simulink model "acc_vm"  (R2025b)
settings: Solver=FixedStepDiscrete  StartTime=0.0  StopTime=10.0  RelTol=1e-3
settings Model: Creator=matthewkeller  LastModifiedBy=ryanj
settings OptimizationCC: DefaultParameterBehavior=Inlined  EnhancedBackFolding=on  PassReuseOutputArgsThreshold=0.0  ZeroExternalMemoryAtStartup=off  ZeroInternalMemoryAtStartup=off  OptimizeBlockOrder=speed  DifferentSizesBufferReuse=on  OptimizationCustomize=off
settings DebuggingCC: ParameterTunabilityLossMsg=error
settings SFSimCC: MATLABDynamicMemAlloc=off
settings RTWCC: SystemTargetFile=rtmaps.tlc  TemplateMakefile=rtmaps_default_tmf  PostCodeGenCommand=rtmaps_post_code_generation(buildInfo)  RetainRTWFile=on  TargetLang=C++  Description=Generate an RTMaps component embedding the model
settings CodeAppCC: ForceParamTrailComments=on  OperatorAnnotations=on
settings STFCustomTargetCC: SystemTargetFile=rtmaps.tlc  TargetLangStandard=C++11 (ISO)  ModelReferenceCompliant=off  CombineOutputUpdateFcns=on  CodeInterfacePackaging=C++ class  SubcomponentCodeInterfacePackaging=C++ class  CPPClassGenCompliant=on  GRTInterface=off  CustomFileTemplate=rtmaps_file_process.tlc  RTMaps_CombineOutputUpdateFcns=1  RTMaps_MatFileLogging=0  DisplayOptimOptions=off  RTMAPS_SDKDIR=C:\Program Files\Intempora\RTMaps 4  RTMAPS_OS=vc.net2022  RTMaps_IntegerCode=0  RTMAPS_BOARD=vc.net2022_x64  RTMaps_GenerateAllocFcn=0  RTMaps_GenerateERTSFunction=0  RTMaps_GRTInterface=0  RTMaps_MultiInstanceCode=1  RTMAPS_ARCH=x86_64
settings GRTTargetCC: TargetLangStandard=C++11 (ISO)  ModelReferenceCompliant=off  ParMdlRefBuildCompliant=off  CompOptLevelCompliant=off  MatFileLogging=off  CodeInterfacePackaging=C++ class  SubcomponentCodeInterfacePackaging=C++ class  UseToolchainInfoCompliant=off

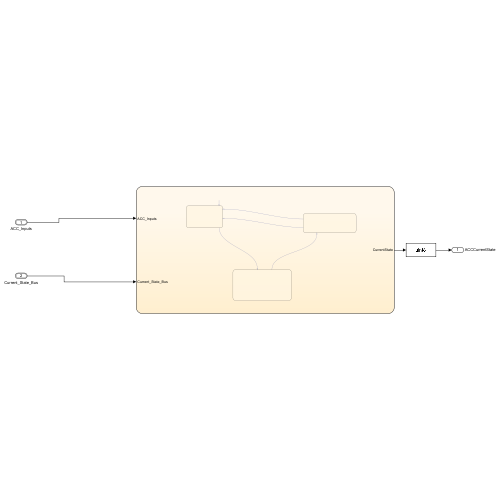
[thumbnail: Simulink's stored preview of the top-level diagram]
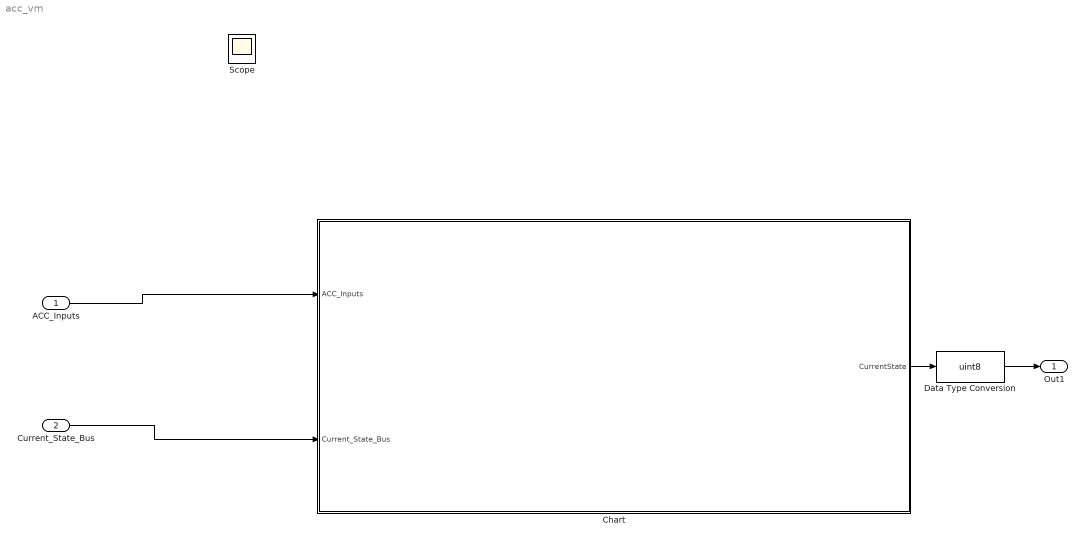
== system acc_vm ==
  ACC_Inputs : Inport  OutDataTypeStr=Bus: ACCStatusBus
  Current_State_Bus : Inport  Port=2  OutDataTypeStr=Bus: CurrentStateBus
  Chart : Stateflow chart  TreatAsAtomicUnit=on
  Data Type Conversion : DataTypeConversion  OutDataTypeStr=uint8  SaturateOnIntegerOverflow=off  RndMeth=Floor
  Out1 : Outport  SignalName=ACCCurrentState
  Scope : Scope
      settings: ActiveDisplayYMinimum=-1  ActiveDisplayYMaximum=1
  wires:
  ACC_Inputs/1 -> Chart/1(ACC_Inputs)
  Current_State_Bus/1 -> Chart/2(Current_State_Bus)
  Chart/1(CurrentState) -> Data Type Conversion/1
  Data Type Conversion/1 -> Out1/1

== stateflow chart acc_vm/Chart ==
  settings: executeAtInitialization=1
  state ACC_Deactivated
    entry:
    CurrentState = StatusType.Deactivated;
  state ACC_Active
    entry:
    CurrentState = StatusType.Active;
  state ACC_Standby
    entry:
    CurrentState = StatusType.Standby;
  (default) -> ACC_Deactivated
  ACC_Active -> ACC_Deactivated [order 2] : [ACC_Inputs.Timeout_Event]
  ACC_Active -> ACC_Deactivated [order 1] : [ACC_Inputs.Cancel_Pressed || ACC_Inputs.Driver_Brakes]
  ACC_Deactivated -> ACC_Standby : [ACC_Inputs.ACC_Enable_Pressed && ACC_Inputs.V2X_Switch_ON && ACC_Inputs.Longitudinal_Switch_ON && Current_State_Bus.APStatus == StatusType.Standby]
  ACC_Standby -> ACC_Active : [ACC_Inputs.Set_Resume && ACC_Inputs.In_CACC_Speed_Range]
  data: ACC_Inputs input Bus: ACCStatusBus; Current_State_Bus input Bus: CurrentStateBus; CurrentState output Enum: StatusType
